simulink library "gap_controller_lib"  (Simulink 8.2)
settings: Solver=ode1  StartTime=0.0  StopTime=Inf  FixedStep=0.001  RelTol=1e-3
PostLoadFcn:
  | , if any(exist('dsrtsu_mdlpostloadfcn', 'file') == [2, 3, 6]), try dsrtsu_mdlpostloadfcn('Execute', bdroot); catch fprintf('Error in PostLoadFcn (dsrtsu_mdlpostloadfcn) for model "%s":\n %s\n', bdroot, lasterr); end, end,
libraries: simulink x2
settings Model: DSRTSU_INTERNAL_RTI_VER=450  DSRTSU_INTERNAL_RTI_TYPE=rti1401  DSRTSU_INTERNAL_RTIFPGA=40  Creator=rushk1  LastModifiedBy=rushk1

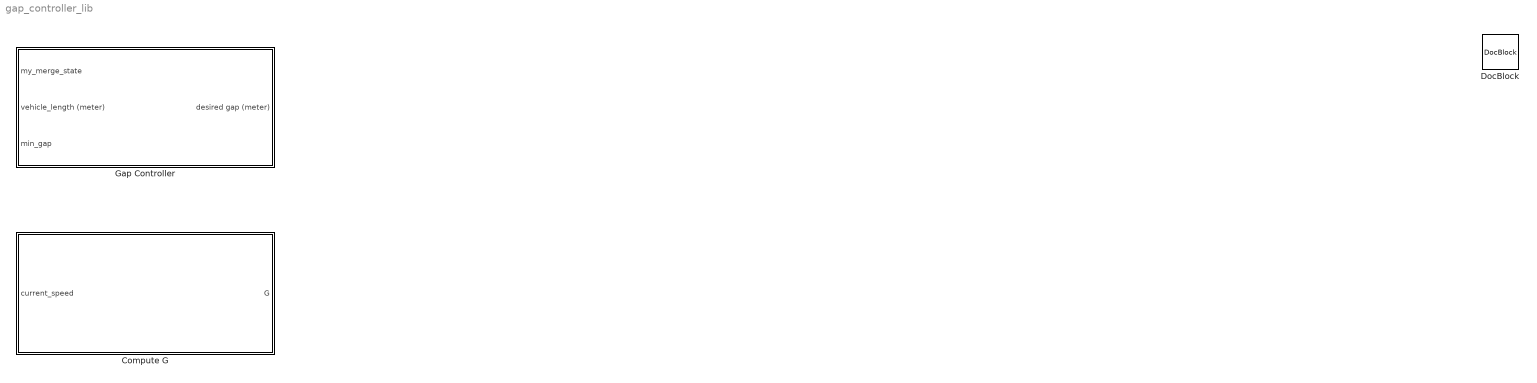
== system gap_controller_lib ==
  Compute G : Subsystem
  DocBlock : simulink/Model-Wide Utilities/DocBlock  DocumentType=Text
      content=|
      | This library is responsible for the desired gap computations.
      |
      | Desired headway between two vehicles is represented as G and is computed as
      | a function of speed. G is computed by determining the distance it the
      | vehicle would need to stop from current speed given some reaction time
      | before braking is applied and some maximum deceleration.
      |
      | This value is used in the determination of merge readiness as well as in
      | gap regulation/speed control.
      |
      | The Gap Controller block determines whether our desired gap is the above
      | mentioned G or 2G + L (where L is vehicle length) when we're trying to make
      | room for the merge vehicle to enter the lane.
  Gap Controller : Subsystem

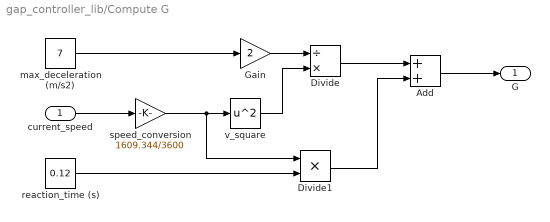
== system gap_controller_lib/Compute G ==
  current_speed : Inport
  Add : Sum
  Divide : Product  Inputs=/*
  Divide1 : Product  Inputs=**
  Gain : Gain  Gain=2
  max_deceleration (m/s2) : Constant  Value=7
  reaction_time (s) : Constant  Value=0.12
  speed_conversion : Gain  Gain=1609.344/3600
  v_square : Math  Operator=square  SaturateOnIntegerOverflow=on
  G : Outport
  wires:
  Divide/1 -> Add/1
  Divide1/1 -> Add/2
  Gain/1 -> Divide/1
  v_square/1 -> Divide/2
  current_speed/1 -> speed_conversion/1
  speed_conversion/1 -> Divide1/1, v_square/1
  max_deceleration (m/s2)/1 -> Gain/1
  reaction_time (s)/1 -> Divide1/2
  Add/1 -> G/1

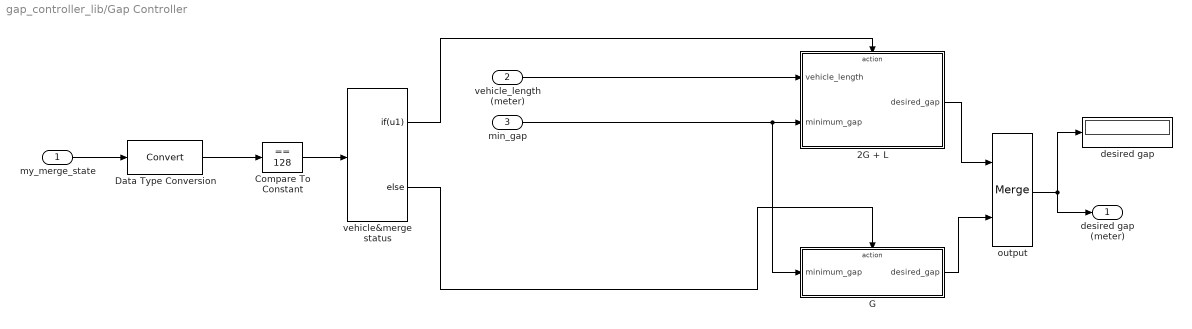
== system gap_controller_lib/Gap Controller ==
  my_merge_state : Inport
  vehicle_length (meter) : Inport  Port=2
  min_gap : Inport  Port=3
  2G + L : Subsystem  TreatAsAtomicUnit=on
  Compare To Constant : simulink/Logic and Bit Operations/Compare To Constant  relop===  const=128  OutDataTypeStr=boolean
  Data Type Conversion : DataTypeConversion
  G : Subsystem  TreatAsAtomicUnit=on
  desired gap : Display
  output : Merge
  vehicle&merge status : If  IfExpression=u1
  desired gap (meter) : Outport
  wires:
  vehicle&merge status/1 -> 2G + L/Action
  vehicle&merge status/2 -> G/Action
  min_gap/1 -> G/1(minimum_gap), 2G + L/2(minimum_gap)
  2G + L/1(desired_gap) -> output/1
  G/1(desired_gap) -> output/2
  output/1 -> desired gap (meter)/1, desired gap/1
  vehicle_length (meter)/1 -> 2G + L/1(vehicle_length)
  my_merge_state/1 -> Data Type Conversion/1
  Compare To Constant/1 -> vehicle&merge status/1
  Data Type Conversion/1 -> Compare To Constant/1

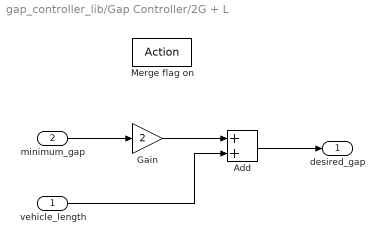
== system gap_controller_lib/Gap Controller/2G + L ==
  vehicle_length : Inport
  minimum_gap : Inport  Port=2
  Merge flag on : ActionPort  ActionType=then
  Add : Sum
  Gain : Gain  Gain=2
  desired_gap : Outport
  wires:
  minimum_gap/1 -> Gain/1
  Gain/1 -> Add/1
  vehicle_length/1 -> Add/2
  Add/1 -> desired_gap/1

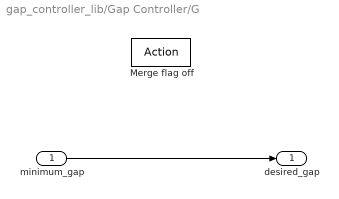
== system gap_controller_lib/Gap Controller/G ==
  minimum_gap : Inport
  Merge flag off : ActionPort  ActionType=else
  desired_gap : Outport
  wires:
  minimum_gap/1 -> desired_gap/1
